simulink model "Aufgabe2_sim"  (R2023b)
settings: Solver=VariableStepAuto  StartTime=0.0  StopTime=20  RelTol=1e-3
values from neighbouring files (symbols this model uses):
  J = 4000e-7    (= 0.0004)    [Aufgabe2_param.m]
  K = 30e-3    (= 0.03)    [Aufgabe2_param.m]
  Kr = Umax/emax    (= 0.1)    [Aufgabe2_param.m]
  L = 120e-6    (= 0.00012)    [Aufgabe2_param.m]
  R = 6    [Aufgabe2_param.m]
settings Model: Creator=rouven  LastModifiedBy=rouven

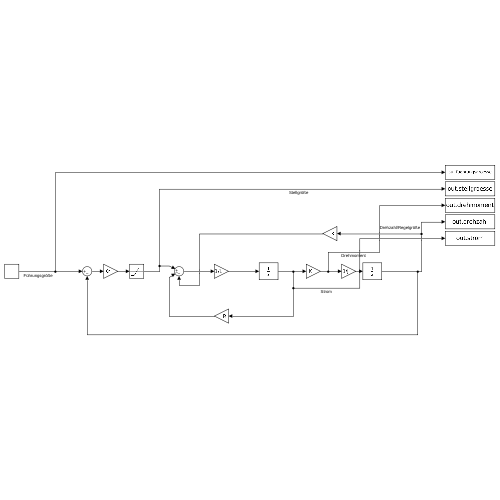
[thumbnail: Simulink's stored preview of the top-level diagram]
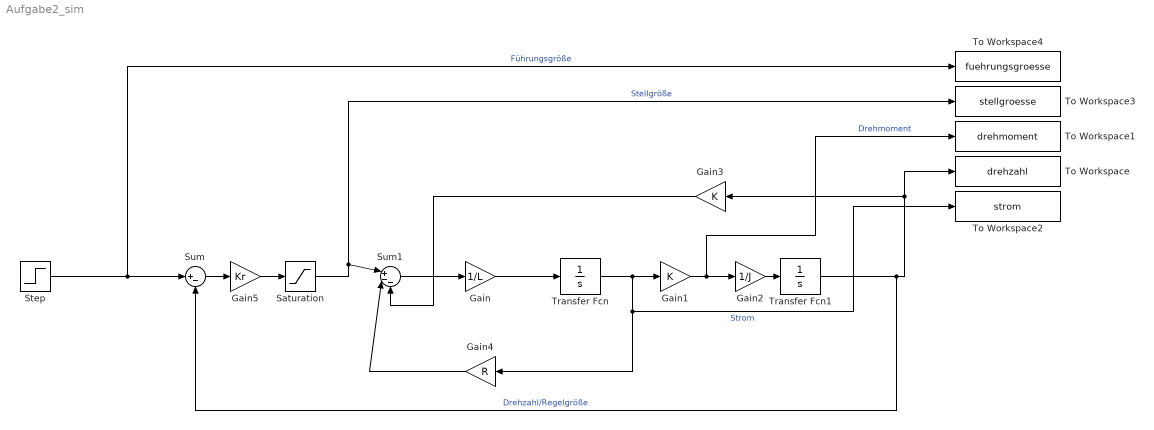
== system Aufgabe2_sim ==
  Gain : Gain  Gain=1/L
  Gain1 : Gain  Gain=K
  Gain2 : Gain  Gain=1/J
  Gain3 : Gain  Gain=K
  Gain4 : Gain  Gain=R
  Gain5 : Gain  Gain=Kr
  Saturation : Saturate  UpperLimit=10  LowerLimit=-10
  Step : Step  After=100  SampleTime=0
  Sum : Sum  Inputs=|+-
  Sum1 : Sum  Inputs=|+--
  To Workspace : ToWorkspace  VariableName=drehzahl  SaveFormat=Structure With Time  SampleTime=-1
  To Workspace1 : ToWorkspace  VariableName=drehmoment  SaveFormat=Structure With Time  SampleTime=-1
  To Workspace2 : ToWorkspace  VariableName=strom  SaveFormat=Structure With Time  SampleTime=-1
  To Workspace3 : ToWorkspace  VariableName=stellgroesse  SaveFormat=Structure With Time  SampleTime=-1
  To Workspace4 : ToWorkspace  VariableName=fuehrungsgroesse  SaveFormat=Structure With Time  SampleTime=-1
  Transfer Fcn : TransferFcn  Denominator=[1 0]
  Transfer Fcn1 : TransferFcn  Denominator=[1 0]
  wires:
  Sum1/1 -> Gain/1
  Gain/1 -> Transfer Fcn/1
  Gain1/1 -> To Workspace1/1, Gain2/1  "Drehmoment"
  Gain2/1 -> Transfer Fcn1/1
  Transfer Fcn1/1 -> Sum/2, To Workspace/1, Gain3/1  "Drehzahl/Regelgröße"
  Transfer Fcn/1 -> To Workspace2/1, Gain4/1, Gain1/1  "Strom"
  Gain4/1 -> Sum1/2
  Gain3/1 -> Sum1/3
  Gain5/1 -> Saturation/1
  Saturation/1 -> To Workspace3/1, Sum1/1  "Stellgröße"
  Step/1 -> To Workspace4/1, Sum/1  "Führungsgröße"
  Sum/1 -> Gain5/1
